simulink model "LQR_inRealTime"  (R2023b)
settings: Solver=VariableStepAuto  StartTime=0.0  StopTime=10.0  RelTol=1e-3
undefined symbols (not defined in the file): A, B, C, D, Discrete, Kr, LF, Time
libraries: svdutilitieslib x3, instrumentseriallib x3, ctrlSharedLib x2, mcbcontrolslib x1
settings Model: Creator=msdbg  LastModifiedBy=msdbg

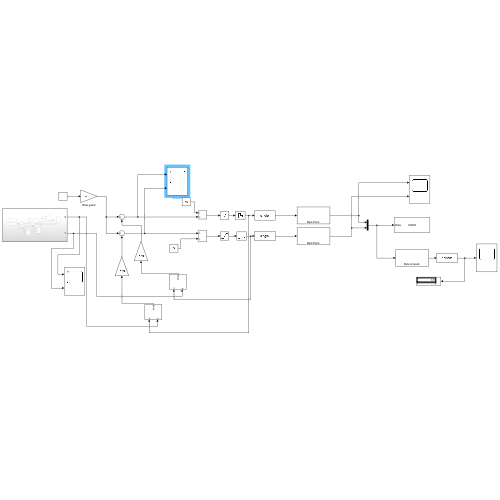
[thumbnail: Simulink's stored preview of the top-level diagram]
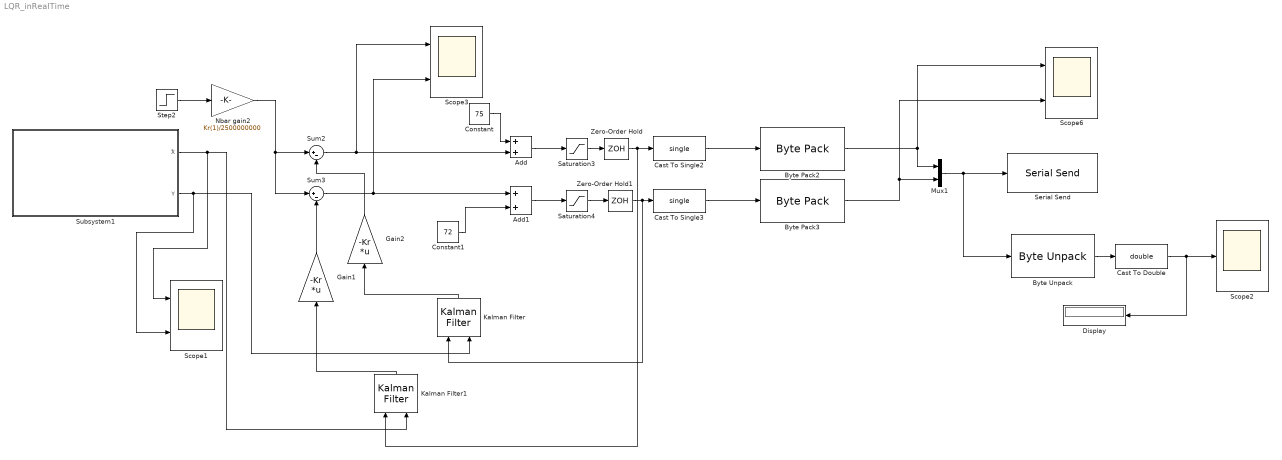
== system LQR_inRealTime ==
  Add : Sum
  Add1 : Sum
  Byte Pack2 : svdutilitieslib/Byte Pack  maskPackedDataType=uint8  datatypes={'single'}  byteAlign=4  blockPlatform=tic2000
      settings: LibrarySourceBlock=c2000lib/Target Communication/Byte Pack
  Byte Pack3 : svdutilitieslib/Byte Pack  maskPackedDataType=uint8  datatypes={'single'}  byteAlign=4  blockPlatform=tic2000
      settings: LibrarySourceBlock=c2000lib/Target Communication/Byte Pack
  Byte Unpack : svdutilitieslib/Byte Unpack  dimensions={[2]}  datatypes={'single'}  byteAlign=4  blockPlatform=tic2000
      settings: LibrarySourceBlock=c2000lib/Target Communication/Byte Unpack
  Cast To Double : DataTypeConversion  OutDataTypeStr=double  SaturateOnIntegerOverflow=off  RndMeth=Floor
  Cast To Single2 : DataTypeConversion  OutDataTypeStr=single  SaturateOnIntegerOverflow=off  RndMeth=Floor
  Cast To Single3 : DataTypeConversion  OutDataTypeStr=single  SaturateOnIntegerOverflow=off  RndMeth=Floor
  Constant : Constant  Value=75
  Constant1 : Constant  Value=72
  Display : Display
  Gain1 : Gain  Gain=-Kr  Multiplication=Matrix(K*u)
  Gain2 : Gain  Gain=-Kr  Multiplication=Matrix(K*u)
  Kalman Filter : ctrlSharedLib/Kalman Filter  TimeDomain=Discrete-Time  UseCurrentEstimator=on  ModelSource=LTI State-Space Variable  ModelSourceVariable=DBPS  A=A  B=B  C=C  D=D  NumberOfStates=1  NumberOfInputs=1  NumberOfOutputs=1  InitialEstimateSource=Dialog  X0=0  P0=10  UseK=off  UseGH=off  NumberOfProcessNoiseInputs=1  G=1  TimeInvariantG=on  H=0  TimeInvariantH=on  Q=w  TimeInvariantQ=on  R=0.01  TimeInvariantR=on  N=0  TimeInvariantN=on  AddInputPort=on  AddEnablePort=off  OutputEstimatedY=off  OutputP=off  Ts=0.05
  Kalman Filter1 : ctrlSharedLib/Kalman Filter  TimeDomain=Discrete-Time  UseCurrentEstimator=on  ModelSource=LTI State-Space Variable  ModelSourceVariable=DBPS  A=A  B=B  C=C  D=D  NumberOfStates=1  NumberOfInputs=1  NumberOfOutputs=1  InitialEstimateSource=Dialog  X0=0  P0=10  UseK=off  UseGH=off  NumberOfProcessNoiseInputs=1  G=1  TimeInvariantG=on  H=0  TimeInvariantH=on  Q=w  TimeInvariantQ=on  R=0.01  TimeInvariantR=on  N=0  TimeInvariantN=on  AddInputPort=on  AddEnablePort=off  OutputEstimatedY=off  OutputP=off  Ts=0.05
  Mux1 : Mux  Inputs=2
  Nbar gain2 : Gain  Gain=Kr(1)/2500000000
  Saturation3 : Saturate  UpperLimit=170  LowerLimit=10
  Saturation4 : Saturate  UpperLimit=170  LowerLimit=10
  Scope1 : Scope  NumInputPorts=2
  Scope2 : Scope
  Scope3 : Scope  NumInputPorts=2
  Scope6 : Scope  NumInputPorts=2
  Serial Send : instrumentseriallib/Serial Send  Priority=1  PortSel=COM3  Port=COM3  ComPort=COM3  Header=[]  Terminator=<none>  CustomTerminator=[]  EnableBlockingMode=on  SimulateUsing=Interpreted execution  BlockInModel=on  aMode=1
  Step2 : Step  Time=0  After=550  SampleTime=0
  Subsystem1 : Subsystem
  Sum2 : Sum  Inputs=|+-
  Sum3 : Sum  Inputs=|+-
  Zero-Order Hold : ZeroOrderHold  SampleTime=0.08
  Zero-Order Hold1 : ZeroOrderHold  SampleTime=0.08
  wires:
  Byte Pack3/1 -> Scope6/2, Mux1/2
  Byte Unpack/1 -> Cast To Double/1
  Saturation3/1 -> Zero-Order Hold/1
  Zero-Order Hold1/1 -> Kalman Filter/1, Cast To Single3/1
  Add/1 -> Saturation3/1
  Sum3/1 -> Add1/1, Scope3/2
  Sum2/1 -> Scope3/1, Add/2
  Constant/1 -> Add/1
  Cast To Single3/1 -> Byte Pack3/1
  Add1/1 -> Saturation4/1
  Cast To Single2/1 -> Byte Pack2/1
  Constant1/1 -> Add1/2
  Saturation4/1 -> Zero-Order Hold1/1
  Mux1/1 -> Byte Unpack/1, Serial Send/1
  Cast To Double/1 -> Display/1, Scope2/1
  Step2/1 -> Nbar gain2/1
  Byte Pack2/1 -> Mux1/1, Scope6/1
  Zero-Order Hold/1 -> Cast To Single2/1, Kalman Filter1/1
  Nbar gain2/1 -> Sum3/1, Sum2/1
  Gain1/1 -> Sum3/2
  Gain2/1 -> Sum2/2
  Kalman Filter/1 -> Gain2/1
  Kalman Filter1/1 -> Gain1/1
  Subsystem1/2(Y) -> Scope1/2, Kalman Filter/2
  Subsystem1/1(ْْX) -> Scope1/1, Kalman Filter1/2

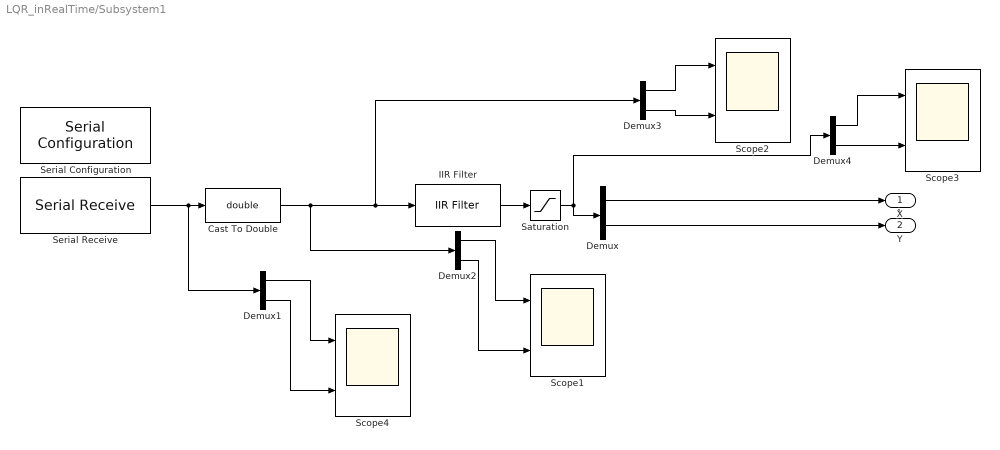
== system LQR_inRealTime/Subsystem1 ==
  Cast To Double : DataTypeConversion  OutDataTypeStr=double  SaturateOnIntegerOverflow=off  RndMeth=Floor
  Demux{,1..4} (5 alike) : Demux  Outputs=2
  IIR Filter : mcbcontrolslib/IIR Filter  VariantControl=Low Pass Filter  VariantSelect=Low-pass  Filter_constant=0.4  advancedSettings=on  Ts=0.05  cutOff_freq=2.1221
      settings: LibrarySourceBlock=mcblib/Signal Management/IIR Filter
  Saturation : Saturate  UpperLimit=800  LowerLimit=300
  Scope{1..4} (4 alike) : Scope  NumInputPorts=2
  Serial Configuration : instrumentseriallib/Serial Configuration  Priority=-200000  PortSel=COM3  Port=COM3  ComPort=COM3  BaudRate=9600  DataBits=8  Parity=none  StopBits=1  ByteOrder=little-endian  FlowControl=none  Timeout=10  SimulateUsing=Interpreted execution  BlockInModel=on  aMode=1
  Serial Receive : instrumentseriallib/Serial Receive  Priority=1  PortSel=COM3  Port=COM3  ComPort=COM3  DataType=single  SaveDataType=uint8  ToggleHeader=on  Header='A'  ToggleTerminator=on  Terminator=LF ('\n')  CustomTerminator=[]  InputFormat=Column major  ToggleDataSize=on  DataSize=[1 2]  EnableBlockingMode=on  ActionDataUnavailable=Output custom value  ActionWhenDataUnavailable=Output custom value  CustomValue=550  SampleTime=0.08  SimulateUsing=Interpreted execution  BlockInModel=on  aMode=1
  ْْX : Outport
  Y : Outport  Port=2
  wires:
  Serial Receive/1 -> Cast To Double/1, Demux1/1
  Demux1/1 -> Scope4/1
  Demux1/2 -> Scope4/2
  Demux2/1 -> Scope1/1
  Demux2/2 -> Scope1/2
  Demux3/1 -> Scope2/1
  Demux3/2 -> Scope2/2
  Demux4/1 -> Scope3/1
  Demux4/2 -> Scope3/2
  Cast To Double/1 -> IIR Filter/1, Demux3/1, Demux2/1
  Demux/1 -> ْْX/1
  Demux/2 -> Y/1
  IIR Filter/1 -> Saturation/1
  Saturation/1 -> Demux4/1, Demux/1
